simulink model "test"  (R2015a)
settings: Solver=ode45  StartTime=0.0  StopTime=100000  RelTol=1e-3
InitFcn:
  | %% DSPBuilder Start
  | alt_dspbuilder_update_model(bdroot)
  | %% DSPBuilder End
libraries: allblocks_alteradspbuilder2 x18
settings Model: Creator=ASUS  LastModifiedBy=ASUS

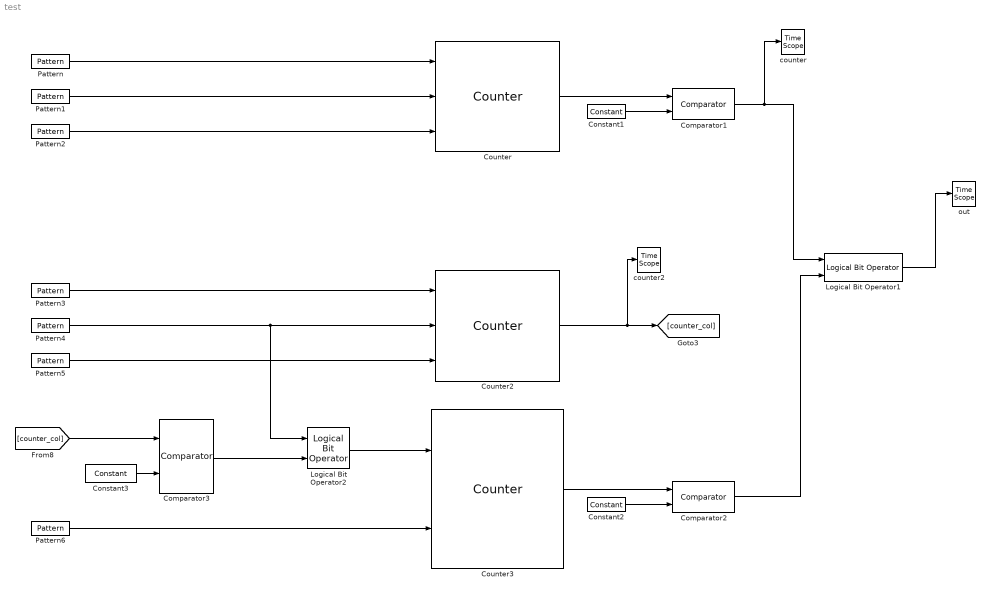
== system test ==
  Comparator1 : allblocks_alteradspbuilder2/Comparator  direction=a == b  pipeline_display=0  allowFloatingPointOverride=on  logOutputs=off  logFile=C:\Users\ASUS\Desktop\sift_fpga_final\Octave_1\tb_test\test_Comparator1.fixedpointlog
  Comparator2 : allblocks_alteradspbuilder2/Comparator  direction=a == b  pipeline_display=0  allowFloatingPointOverride=on  logOutputs=off  logFile=C:\Users\ASUS\Desktop\sift_fpga_final\Octave_1\tb_test\test_Comparator2.fixedpointlog
  Comparator3 : allblocks_alteradspbuilder2/Comparator  direction=a == b  pipeline_display=0  allowFloatingPointOverride=on  logOutputs=off  logFile=C:\Users\ASUS\Desktop\sift_fpga_final\Octave_1\tb_test\test_Comparator3.fixedpointlog
  Constant1 : allblocks_alteradspbuilder2/Constant  mask_cst=1  BusType=Unsigned Integer  bwl=2  bwr=0  roundMode=Truncate  satMode=Wrap  SpecifyClock=off  allowFloatingPointOverride=on  logOutputs=off  logFile=C:\Users\ASUS\Desktop\sift_fpga_final\Octave_1\tb_test\test_Constant1.fixedpointlog
  Constant2 : allblocks_alteradspbuilder2/Constant  mask_cst=0  BusType=Unsigned Integer  bwl=2  bwr=0  roundMode=Truncate  satMode=Wrap  SpecifyClock=off  allowFloatingPointOverride=on  logOutputs=off  logFile=C:\Users\ASUS\Desktop\sift_fpga_final\Octave_1\tb_test\test_Constant2.fixedpointlog
  Constant3 : allblocks_alteradspbuilder2/Constant  mask_cst=639  BusType=Unsigned Integer  bwl=10  bwr=0  roundMode=Truncate  satMode=Wrap  SpecifyClock=off  allowFloatingPointOverride=on  logOutputs=off  logFile=C:\Users\ASUS\Desktop\sift_fpga_final\Octave_1\tb_test\test_Constant3.fixedpointlog
  Counter : allblocks_alteradspbuilder2/Counter  BusType=Unsigned Integer  bwl=2  bwr=0  use_modulo=on  modulo=2  SpecifyClock=off  direction=Increment  use_sload=off  use_sset=on  svalue=0  use_clk_ena=off  use_ena=on  use_sclr=on  pipeline_display=1
  Counter2 : allblocks_alteradspbuilder2/Counter  BusType=Unsigned Integer  bwl=10  bwr=0  use_modulo=on  modulo=640  SpecifyClock=off  direction=Increment  use_sload=off  use_sset=on  svalue=0  use_clk_ena=off  use_ena=on  use_sclr=on  pipeline_display=1
  Counter3 : allblocks_alteradspbuilder2/Counter  BusType=Unsigned Integer  bwl=2  bwr=0  use_modulo=on  modulo=2  SpecifyClock=off  direction=Increment  use_sload=off  use_sset=off  svalue=0  use_clk_ena=off  use_ena=on  use_sclr=on  pipeline_display=1
  Logical Bit Operator1 : allblocks_alteradspbuilder2/Logical Bit Operator  LogicalOperator=AND  user_inputs=2  pipeline_display=0
  Logical Bit Operator2 : allblocks_alteradspbuilder2/Logical Bit Operator  LogicalOperator=AND  user_inputs=2  pipeline_display=0
  Pattern : allblocks_alteradspbuilder2/Pattern  Sequence=0001000010000100001000010000  SpecifyClock=off  use_ena=off  use_sclr=off
  Pattern1 : allblocks_alteradspbuilder2/Pattern  Sequence=111111111111111111111111111111  SpecifyClock=off  use_ena=off  use_sclr=off
  Pattern2 : allblocks_alteradspbuilder2/Pattern  Sequence=0010000100001000010000100001  SpecifyClock=off  use_ena=off  use_sclr=off
  Pattern3 : allblocks_alteradspbuilder2/Pattern  Sequence=0001000010000100001000010000  SpecifyClock=off  use_ena=off  use_sclr=off
  Pattern4 : allblocks_alteradspbuilder2/Pattern  Sequence=111111111111111111111111111111  SpecifyClock=off  use_ena=off  use_sclr=off
  Pattern5 : allblocks_alteradspbuilder2/Pattern  Sequence=0010000100001000010000100001  SpecifyClock=off  use_ena=off  use_sclr=off
  Pattern6 : allblocks_alteradspbuilder2/Pattern  Sequence=0010000100001000010000100001  SpecifyClock=off  use_ena=off  use_sclr=off
  counter : TimeScope  DefaultConfigurationName=spbscopes.TimeScopeBlockCfg
  counter2 : TimeScope  DefaultConfigurationName=spbscopes.TimeScopeBlockCfg
  out : TimeScope  DefaultConfigurationName=spbscopes.TimeScopeBlockCfg
  wires:
  Counter3/1 -> Comparator2/1
  Counter/1 -> Comparator1/1
  Pattern1/1 -> Counter/2
  Constant1/1 -> Comparator1/2
  Comparator1/1 -> counter/1, Logical Bit Operator1/1
  Pattern2/1 -> Counter/3
  Constant2/1 -> Comparator2/2
  Comparator2/1 -> Logical Bit Operator1/2
  Logical Bit Operator1/1 -> out/1
  Pattern6/1 -> Counter3/2
  Logical Bit Operator2/1 -> Counter3/1
  [counter_col] -> Comparator3/1
  Constant3/1 -> Comparator3/2
  Comparator3/1 -> Logical Bit Operator2/2
  Pattern4/1 -> Counter2/2, Logical Bit Operator2/1
  Pattern5/1 -> Counter2/3
  Pattern/1 -> Counter/1
  Pattern3/1 -> Counter2/1
  Counter2/1 -> counter2/1, [counter_col]
